simulink library "servoLibrary"  (R2019a)
settings: Solver=VariableStepAuto  StartTime=0.0  StopTime=10.0  RelTol=1e-3
undefined symbols (not defined in the file): etaMask, gearRatioMask, JMask, rpm0Mask, rpm_etaMask, rpm_maxMask, T_iMask, trq_etaMask, trq_stallMask
libraries: nesl_utility x3, fl_lib x2, ee_lib x1
Description:
  | Copyright 2008-2019 The MathWorks, Inc.
  | 
  | Servo library
settings Model: Creator=falderis  LastModifiedBy=falderis
settings DataIOCC: ReturnWorkspaceOutputs=off
settings DebuggingCC: ArithmeticOperatorsInVariantConditions=warning

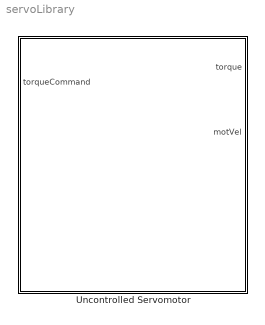
== system servoLibrary ==
  Uncontrolled Servomotor : Subsystem  Tag=PublishSubsystem  mask(Servomotor){T_i=T_iMask, eta=etaMask, rpm_eta=rpm_etaMask, trq_eta=trq_etaMask, trq_stall=trq_stallMask, rpm_max=rpm_maxMask, J=JMask, rpm0=rpm0Mask, gearRatio=gearRatioMask}
      mask prompts: T_i "Current loop time constant (s)"; eta "Efficiency (%)"; rpm_eta "Speed at which efficiency measured (rpm)"; trq_eta "Torque at which efficiency measured  (Nm)"; trq_stall "Stall torque (Nm)"; rpm_max "Maximum speed (rpm)"; J "Rotor inertia (kg*m^2)"; rpm0 "Rotor initial speed (rpm)"; gearRatio "Gearbox ratio"
      mask help: Implements an abstracted model of a servomotor.
      mask DialogControl ParameterTabVar0 Prompt: Electrical
      mask DialogControl ParameterTabVar01 Prompt: Efficiency
      mask DialogControl ParameterTabVar012 Prompt: Mechanical

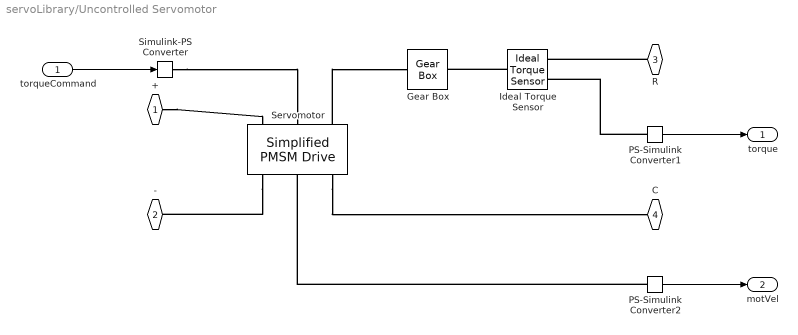
== system servoLibrary/Uncontrolled Servomotor ==
  torqueCommand : Inport
  Gear Box : fl_lib/Mechanical/Mechanisms/Gear Box  ratio=gearRatio  t_in_specify=off  t_in_priority=None  t_in=0 N*m  t_in_nominal_specify=off  t_in_nominal_unit=N*m  t_in_nominal_value=1  t_out_specify=off  t_out_priority=None  t_out=0 N*m  t_out_nominal_specify=off  t_out_nominal_unit=N*m  t_out_nominal_value=1
  Ideal Torque Sensor : fl_lib/Mechanical/Mechanical Sensors/Ideal Torque Sensor
  PS-Simulink Converter1 : nesl_utility/PS-Simulink Converter  PhysicalDomain=network_engine_domain  SubClassName=ps_output  LeftPortType=input  RightPortType=output  PseudoPeriodic=off  Frequencies=[]  Unit=N*m  AffineConversion=off
  PS-Simulink Converter2 : nesl_utility/PS-Simulink Converter  PhysicalDomain=network_engine_domain  SubClassName=ps_output  LeftPortType=input  RightPortType=output  PseudoPeriodic=off  Frequencies=[]  Unit=rpm  AffineConversion=off
  Servomotor : ee_lib/Electromechanical/Permanent Magnet/Simplified PMSM Drive  torque_speed_param=1  w_t=[0 0.98 0.99 1] * rpm_max rpm  T_t=[1 1 1 0] * trq_stall N*m  torque_max=0.1 N*m  power_max=30 W  Tc=T_i s  losses_param=1  eff=eta  w_eff=rpm_eta rpm  T_eff=trq_eta N*m  Piron=0 W  Pbase=0 W  w_eff_vec=[-8000 -4000 0 4000 8000] rpm  T_eff_vec=[0 0.03 0.06 0.09] N*m  v_eff_vec=[100, 250, 400] V  losses_mat=[1.49 1.67 2.21 3.10; 0.42 0.69 1.14 2.03; 0.06 0.24 0.78 1.68; 0.42 0.69 1.14 2.03; 1.49 1.67 2.21 3.10] W  efficiency_mat=[95 95 95 95; 95 95 95 95; 95 95 95 95; 95 95 95 95; 95 95 95 95]  losses_mat_3D=ones(5, 4, 3) W  efficiency_mat_3D=95 * ones(5, 4, 3)  Res=0 Ohm  J=J kg*m^2  lam=0 N*m/(rad/s)  speed0=rpm0 rpm  faulted_specify=off  faulted_priority=None  faulted=0  faulted_nominal_specify=off  faulted_nominal_unit=1  faulted_nominal_value=1  alpha=3.93e-3 1/K  Tmeas=25 degC  Tmeas2=125 degC  losses_mat_T2=[1.49, 1.74, 2.49, 3.74; .42, .67, 1.42, 2.67; .06, .31, 1.06, 2.31; .42, .67, 1.42, 2.67; 1.49, 1.74, 2.49, 3.74] W  efficiency_mat_T2=[95, 95, 95, 95; 95, 95, 95, 95; 95, 95, 95, 95; 95, 95, 95, 95; 95, 95, 95, 95]  losses_mat_3D_T2=ones(5, 4, 3) W  efficiency_mat_3D_T2=95 * ones(5, 4, 3)  thermal_mass=100 J/K  initial_temperature=25 degC  fault_condition=1  fault_threshold=0.5
      settings: SourceProductName=Simscape Electrical  SourceProductBaseCode=PS
  Simulink-PS Converter : nesl_utility/Simulink-PS Converter  PhysicalDomain=network_engine_domain  SubClassName=ps_input  LeftPortType=input  RightPortType=output  PseudoPeriodic=off  Frequencies=[]  NoiseDistribution=none  NoiseParameters=[]  Unit=N*m  AffineConversion=off  FilteringAndDerivatives=filter  SimscapeFilterOrder=2  InputFilterTimeConstant=0.001  UdotUserProvided=0
  + : PMIOPort  Side=Left
  - : PMIOPort  Port=2  Side=Left
  R : PMIOPort  Port=3  Side=Right
  C : PMIOPort  Port=4  Side=Right
  torque : Outport
  motVel : Outport  Port=2  Unit=rpm
  wires:
  PS-Simulink Converter1/1 -> torque/1
  PS-Simulink Converter2/1 -> motVel/1
  torqueCommand/1 -> Simulink-PS Converter/1
  connections:
  Simulink-PS Converter/RConn1 -- Servomotor/LConn2
  Servomotor/RConn3 -- C/RConn1
  Servomotor/RConn1 -- -/RConn1
  Servomotor/LConn3 -- Gear Box/LConn1
  +/RConn1 -- Servomotor/LConn1
  Ideal Torque Sensor/LConn1 -- Gear Box/RConn1
  R/RConn1 -- Ideal Torque Sensor/RConn1
  PS-Simulink Converter1/LConn1 -- Ideal Torque Sensor/RConn2
  PS-Simulink Converter2/LConn1 -- Servomotor/RConn2
